simulink model "State_machine"  (R2023b)
settings: Solver=VariableStepAuto  StartTime=0.0  StopTime=10.0  RelTol=1e-3
settings Model: Creator=Moisa Versatu  LastModifiedBy=Moisa Versatu

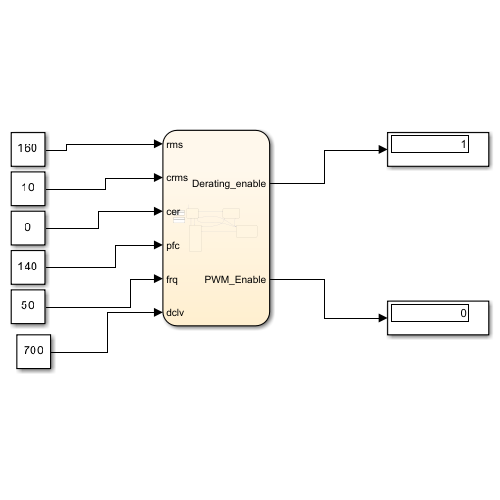
[thumbnail: Simulink's stored preview of the top-level diagram]
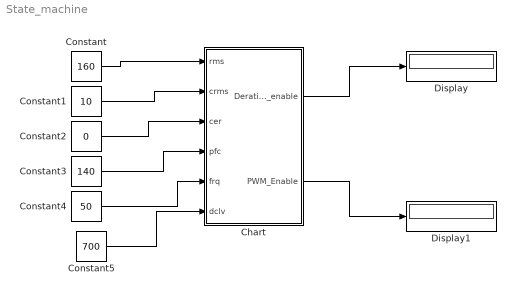
== system State_machine ==
  Chart : Stateflow chart  TreatAsAtomicUnit=on
  Constant : Constant  Value=160
  Constant1 : Constant  Value=10
  Constant2 : Constant  Value=0
  Constant3 : Constant  Value=140
  Constant4 : Constant  Value=50
  Constant5 : Constant  Value=700
  Display : Display
  Display1 : Display
  wires:
  Constant4/1 -> Chart/5(frq)
  Constant3/1 -> Chart/4(pfc)
  Constant2/1 -> Chart/3(cer)
  Constant1/1 -> Chart/2(crms)
  Constant/1 -> Chart/1(rms)
  Chart/2(PWM_Enable) -> Display1/1
  Chart/1(Derating_enable) -> Display/1
  Constant5/1 -> Chart/6(dclv)

== stateflow chart State_machine/Chart ==
  state Idle
    entry:
    flag1 = f(rms,frq,cer,pfc,crms);
    flag = f1(rms,frq,dclv,pfc,crms);
    during:
    if pfc>120
    Derating_enable=1;
    end
    flag1 = f(rms,frq,cer,pfc,crms);
    flag = f1(rms,frq,dclv,pfc,crms);
  state Pre_charge
    entry:
    flag1 = f(rms,frq,cer,pfc,crms);
    flag = f1(rms,frq,dclv,pfc,crms);
    during:
    if pfc>120
    Derating_enable=1;
    end
    flag1 = f(rms,frq,cer,pfc,crms);
  state Error
    entry:
    if flag==2
    fprintf('AC Undervoltage')
    end
    if flag==3
    fprintf('AC Overvoltage')
    end
    if flag==4
    fprintf('Underfrequency')
    end
    if flag==5
    fprintf('Overfrequency')
    end
    if flag==6
    fprintf('DC Link Undervoltage')
    end
    if flag==7
    fprintf('DC Link Overvoltage')
    end
    if flag==8
    fprintf('PFC Overheated')
    end
    if flag==9
    fprintf('AC Overcurrent')
    end
    during:
    flag = f1(rms,frq,dclv,pfc,crms)
  state Charging
    entry:
    flag = f(rms,frq,cer,pfc,crms);
    flag1 = f1(rms,frq,dclv,pfc,crms);
    during:
    if pfc>120
    Derating_enable=1;
    end
    flag = f(rms,frq,cer,pfc,crms);
    flag1 = f1(rms,frq,dclv,pfc,crms);
  (default) -> Idle
  Idle -> Pre_charge [order 1] : [flag1==1 && dclv<=400 ]
  Charging -> Idle [order 2] : [cer==1]
  Pre_charge -> Error [order 2] : [flag==0]
  Pre_charge -> Charging [order 1] : [flag1==1 && dclv>=600 && dclv<=800 && after(2,sec)]{PWM_Enable=1}
  Error -> Idle : [after(2,sec)]
  Idle -> Error [order 3] : [flag==0]
  Idle -> Charging [order 2] : [flag1==1 && dclv>=600 && dclv<=800]{PWM_Enable=1}
  Charging -> Error [order 1] : [flag==0]
  data: rms function_input; frq function_input; cer function_input; pfc function_input; crms function_input; flag1 function_output; rms function_input; frq function_input; dclv function_input; pfc function_input; crms function_input; flag function_output; Derating_enable output; rms input; crms input; cer input; pfc input; frq input; PWM_Enable output; dclv input; flag1 local; flag local
  function flag1 = f(rms,frq,cer,pfc,crms):
    | function flag1 = f(rms,frq,cer,pfc,crms)
    | flag1=1;
    | if rms<185 || rms>265
    |     flag1=0;
    | end
    | if frq<45 || frq>65
    |     flag1=0;
    | end
    | if cer~=0
    |     flag1=0;
    | end
    | if pfc>150
    |     flag1=0;
    | end
    | if crms>16
    |     flag1=0;
    | end
    | end
  function flag = f1(rms,frq,dclv,pfc,crms):
    | function flag = f1(rms,frq,dclv,pfc,crms)
    | flag=0;
    | if rms<185
    |     flag=2;
    | end
    | if rms>265
    |     flag=3;
    | end
    | if frq<45
    |     flag=4;
    | end
    | if frq>65
    |     flag=5;
    | end
    | if dclv<600
    |     flag=6;
    | end
    | if dclv>800
    |     flag=7;
    | end
    | if pfc>150
    |     flag=8;
    | end
    | if crms>16
    |     flag=9;
    | end
    | end
